simulink model "SGBMDisparity"  (R2021a)
settings: Solver=FixedStepDiscrete  StartTime=0.0  StopTime=simT  FixedStep=1  RelTol=1e-3
PreLoadFcn:
  | DL128 = Simulink.Variant('disparityLevels==128');
  | 
  | DLnot128 = Simulink.Variant('disparityLevels ~= 128');
  | 
  | disparityLevels = 64;
  | 
  | imgRowSize = 480;
  | 
  | imgColSize = 640;
  | 
  | P2 = 200; % Smoothness Penalty Large
  | P1 = 15;  % Smoothness Penalty Small
  | 
  | disparityFactor = 16;
  | 
  | uniquenessRatio = 5;
  | 
  | p = imgColSize - 1;
  | q = imgRowSize * imgColSize -1;
  | r = imgColSize - disparityLevels -1;
  | s = (imgRowSize*(imgColSize-disparityLevels))-1;
  | 
  | simT = 800*525
  | 
  | dtGain = 4;
InitFcn:
  | DL128 = Simulink.Variant('disparityLevels==128');
  | 
  | DLnot128 = Simulink.Variant('disparityLevels ~= 128');
  | 
  | img = imread(get_param('SGBMDisparity/stereoImage','FileName'));
  | 
  | [imgRowSize, imgColSize,chn] = size(img);
  | 
  | P2 = 200; % Smoothness Penalty Large
  | P1 = 15;  % Smoothness Penalty Small
  | 
  | disparityFactor = 16;
  | 
  | uniquenessRatio = str2num(get_param('SGBMDisparity/SGBMHDLAlgorithm/SGBMHDLAlgorithmWorker','UT'));
  | 
  | disparityLevels = str2num(get_param('SGBMDisparity/SGBMHDLAlgorithm/SGBMHDLAlgorithmWorker','DL'));
  | 
  | p = imgColSize - 1;
  | q = imgRowSize * imgColSize -1;
  | r = imgColSize - disparityLevels -1;
  | s = (imgRowSize*(imgColSize-disparityLevels))-1;
  | 
  | if imgRowSize == 720 && imgColSize == 1280
  | simT = 1650*750;
  | elseif imgRowSize == 540 && imgColSize == 960
  | simT = 1050*600;
  | elseif imgRowSize == 480 && imgColSize == 640
  | simT = 800*525;
  | end
  | 
  | %if imgRowSize == 720 && imgColSize == 1280
  | %dtGain = 2;
  | %elseif imgRowSize == 540 && imgColSize == 960
  | %dtGain = 2.6;
  | %elseif imgRowSize == 480 && imgColSize == 640
  | %dtGain = 4;
  | %end
  | 
  | dtGain = 8;
libraries: simulink x331, hdlsllib x113, visionhdlutilities x9, visionhdlio x2, visionsources x1
(part 2 of 6)

== system SGBMDisparity/SGBMHDLAlgorithm/SGBMHDLAlgorithmWorker/DirectionalCost/RightToLeft/InverseRow_ForEach ==
  In : Inport  Partition=on  PartitionDimension=1  PartitionWidth=1  PartitionOffset=0
  busIn : Inport  Port=2
  Bus Selector : BusSelector  OutputSignals=valid,hStart,hEnd,vStart
  Compare To Constant : simulink/Logic and Bit Operations/Compare To Constant  relop===  const=1  OutDataTypeStr=boolean
  Compare To Constant1 : simulink/Logic and Bit Operations/Compare To Constant  relop===  const=1  OutDataTypeStr=boolean
  Compare To Constant3 : simulink/Logic and Bit Operations/Compare To Constant  relop===  const=1  OutDataTypeStr=boolean
  Compare To Constant4 : simulink/Logic and Bit Operations/Compare To Constant  relop===  const=imgColSize-disparityLevels-1  OutDataTypeStr=boolean
  Constant : Constant  Value=0  OutDataTypeStr=boolean  SampleTime=-1
  Constant1 : Constant  Value=0  OutDataTypeStr=boolean  SampleTime=-1
  Delay{1..8} (8 alike) : Delay  DelayLength=1
  For Each : ForEach  DisableCoverage=on
  HDL Counter : hdlsllib/Sources/HDL Counter  CountType=Count limited  CountInit=0  CountStep=1  CountMax=imgColSize-disparityLevels-1  CountFromType=Initial value  CountFrom=0  CountResetPort=on  CountLoadPort=off  CountEnbPort=on  CountDirPort=off  CountHitOutputPort=off  CountDataType=Unsigned  CountWordLen=ceil(log2(imgColSize-disparityLevels-1))  CountFracLen=0  CountSampTime=1
  HDL Counter1 : hdlsllib/Sources/HDL Counter  CountType=Count limited  CountInit=imgColSize-disparityLevels-1  CountStep=1  CountMax=0  CountFromType=Initial value  CountFrom=imgColSize-disparityLevels-1  CountResetPort=on  CountLoadPort=off  CountEnbPort=on  CountDirPort=on  CountHitOutputPort=off  CountDataType=Unsigned  CountWordLen=ceil(log2(imgColSize-disparityLevels-1))  CountFracLen=0  CountSampTime=1
  HDL Counter2 : hdlsllib/Sources/HDL Counter  CountType=Count limited  CountInit=0  CountStep=1  CountMax=1  CountFromType=Initial value  CountFrom=0  CountResetPort=on  CountLoadPort=off  CountEnbPort=on  CountDirPort=off  CountHitOutputPort=off  CountDataType=Unsigned  CountWordLen=1  CountFracLen=0  CountSampTime=1
  HDL Counter3 : hdlsllib/Sources/HDL Counter  CountType=Count limited  CountInit=imgColSize-disparityLevels-1  CountStep=1  CountMax=0  CountFromType=Initial value  CountFrom=imgColSize-disparityLevels-1  CountResetPort=on  CountLoadPort=off  CountEnbPort=on  CountDirPort=on  CountHitOutputPort=off  CountDataType=Unsigned  CountWordLen=ceil(log2(imgColSize-disparityLevels-1))  CountFracLen=0  CountSampTime=1
  HDL Counter4 : hdlsllib/Sources/HDL Counter  CountType=Count limited  CountInit=0  CountStep=1  CountMax=imgColSize-disparityLevels-1  CountFromType=Initial value  CountFrom=0  CountResetPort=on  CountLoadPort=off  CountEnbPort=on  CountDirPort=off  CountHitOutputPort=off  CountDataType=Unsigned  CountWordLen=ceil(log2(imgColSize-disparityLevels-1))  CountFracLen=0  CountSampTime=1
  HDL Counter5 : hdlsllib/Sources/HDL Counter  CountType=Count limited  CountInit=0  CountStep=1  CountMax=1  CountFromType=Initial value  CountFrom=0  CountResetPort=on  CountLoadPort=off  CountEnbPort=on  CountDirPort=off  CountHitOutputPort=off  CountDataType=Unsigned  CountWordLen=1  CountFracLen=0  CountSampTime=1
  HDL Counter6 : hdlsllib/Sources/HDL Counter  CountType=Count limited  CountInit=0  CountStep=1  CountMax=imgColSize-disparityLevels-1  CountFromType=Initial value  CountFrom=0  CountResetPort=on  CountLoadPort=off  CountEnbPort=on  CountDirPort=off  CountHitOutputPort=off  CountDataType=Unsigned  CountWordLen=ceil(log2(imgColSize-disparityLevels-1))  CountFracLen=0  CountSampTime=1
  HDL Counter7 : hdlsllib/Sources/HDL Counter  CountType=Count limited  CountInit=0  CountStep=1  CountMax=1  CountFromType=Initial value  CountFrom=0  CountResetPort=on  CountLoadPort=off  CountEnbPort=on  CountDirPort=off  CountHitOutputPort=off  CountDataType=Unsigned  CountWordLen=2  CountFracLen=0  CountSampTime=1
  Logical Operator : Logic  AllPortsSameDT=off  OutDataTypeStr=boolean
  Logical Operator1 : Logic  Operator=OR  AllPortsSameDT=off  OutDataTypeStr=boolean
  Rd_En : simulink/Logic and Bit Operations/Compare To Constant  relop=<=  const=imgColSize-disparityLevels-1  OutDataTypeStr=boolean
  Simple Dual Port RAM : hdlsllib/HDL RAMs/Simple Dual Port RAM  ram_size=ceil(log2(imgColSize-disparityLevels-1))
      settings: SourceProductBaseCode=SL
  Switch : Switch  Criteria=u2 ~= 0
  Switch1 : Switch  Criteria=u2 ~= 0
  Out : Outport  ConcatenationDimension=1  VectorParamsAs1DForOutWhenUnconnected=off
  valid_Out : Outport  Port=2  ConcatenationDimension=1  VectorParamsAs1DForOutWhenUnconnected=off
  wires:
  Compare To Constant4/1 -> Logical Operator1/2, HDL Counter6/1
  Simple Dual Port RAM/1 -> Out/1
  In/1 -> Delay4/1
  Delay7/1 -> valid_Out/1
  Constant/1 -> HDL Counter1/3
  Logical Operator/1 -> HDL Counter4/2, Delay7/1, HDL Counter3/2
  Compare To Constant/1 -> Switch/2
  Rd_En/1 -> Logical Operator/2
  HDL Counter2/1 -> Compare To Constant/1
  Switch1/1 -> Simple Dual Port RAM/4
  HDL Counter4/1 -> Switch1/3
  Compare To Constant1/1 -> Switch1/2
  HDL Counter/1 -> Switch/1
  Delay3/1 -> HDL Counter7/2, HDL Counter5/2
  HDL Counter7/1 -> Compare To Constant3/1
  Constant1/1 -> HDL Counter3/3
  Delay1/1 -> Simple Dual Port RAM/3, HDL Counter1/2, HDL Counter/2
  HDL Counter6/1 -> Rd_En/1, Compare To Constant4/1
  Compare To Constant3/1 -> Logical Operator/1, HDL Counter6/2
  HDL Counter3/1 -> Switch1/1
  Switch/1 -> Simple Dual Port RAM/2
  HDL Counter5/1 -> Compare To Constant1/1
  HDL Counter1/1 -> Switch/3
  Delay2/1 -> Simple Dual Port RAM/1
  Bus Selector/1 -> Delay5/1  "<valid>"
  busIn/1 -> Bus Selector/1
  Bus Selector/2 -> Delay6/1  "<hStart>"
  Bus Selector/3 -> Delay8/1  "<hEnd>"
  Logical Operator1/1 -> HDL Counter7/1
  Bus Selector/4 -> Logical Operator1/1, HDL Counter5/1, HDL Counter2/1, HDL Counter4/1, HDL Counter3/1, HDL Counter/1, HDL Counter1/1  "<vStart>"
  Delay4/1 -> Delay2/1
  Delay5/1 -> Delay1/1
  Delay6/1 -> HDL Counter2/2
  Delay8/1 -> Delay3/1

== system SGBMDisparity/SGBMHDLAlgorithm/SGBMHDLAlgorithmWorker/DirectionalCost/RightToLeft/pixelBusGenerator ==
  validIn : Inport
  Horizontal : hdlsllib/Sources/HDL Counter  CountType=Count limited  CountInit=0  CountStep=1  CountMax=hEnd  CountFromType=Initial value  CountFrom=0  CountResetPort=off  CountLoadPort=off  CountEnbPort=on  CountDirPort=off  CountHitOutputPort=off  CountDataType=Unsigned  CountWordLen=ceil(log2(hEnd))  CountFracLen=0  CountSampTime=1
  Logical Operator{3..6} (4 alike) : Logic  AllPortsSameDT=off  OutDataTypeStr=boolean
  Pixel Control Bus Creator : visionhdlutilities/Pixel Control Bus Creator
      settings: SourceProductBaseCode=VT
  Vertical : hdlsllib/Sources/HDL Counter  CountType=Count limited  CountInit=0  CountStep=1  CountMax=vEnd  CountFromType=Initial value  CountFrom=0  CountResetPort=off  CountLoadPort=off  CountEnbPort=on  CountDirPort=off  CountHitOutputPort=off  CountDataType=Unsigned  CountWordLen=ceil(log2(vEnd))  CountFracLen=0  CountSampTime=1
  hEnd : simulink/Logic and Bit Operations/Compare To Constant  relop===  const=hEnd  OutDataTypeStr=boolean
  hStart : simulink/Logic and Bit Operations/Compare To Constant  relop===  const=0  OutDataTypeStr=boolean
  vEnd : simulink/Logic and Bit Operations/Compare To Constant  relop===  const=vEnd  OutDataTypeStr=boolean
  vStart : simulink/Logic and Bit Operations/Compare To Constant  relop===  const=0  OutDataTypeStr=boolean
  busOut : Outport  VectorParamsAs1DForOutWhenUnconnected=off
  wires:
  validIn/1 -> Pixel Control Bus Creator/5, Vertical/1, Logical Operator4/1, Logical Operator5/1, Logical Operator6/1, Logical Operator3/1, Horizontal/1
  Horizontal/1 -> hEnd/1, hStart/1
  hEnd/1 -> Logical Operator4/2
  Vertical/1 -> vStart/1, vEnd/1
  vStart/1 -> Logical Operator5/2
  vEnd/1 -> Logical Operator6/2
  Logical Operator5/1 -> Pixel Control Bus Creator/3
  Logical Operator3/1 -> Pixel Control Bus Creator/1
  Logical Operator4/1 -> Pixel Control Bus Creator/2
  hStart/1 -> Logical Operator3/2
  Logical Operator6/1 -> Pixel Control Bus Creator/4
  Pixel Control Bus Creator/1 -> busOut/1

== system SGBMDisparity/SGBMHDLAlgorithm/SGBMHDLAlgorithmWorker/DirectionalCost/RightToLeft/rlSubsystem ==
  enable : Inport
  matchCostIn : Inport  Port=2
  Enable : EnablePort
  Delay : Delay  DelayLength=1
  For Each Subsystem : Subsystem  TreatAsAtomicUnit=on
  MinMax1 : MinMax  ZeroCross=off
  Signal Specification : SignalSpecification  Dimensions=disparityLevels
  Switch32 : Switch  Criteria=u2 ~= 0
  d+1 : Subsystem
  d-1 : Subsystem
  minCostPath : Subsystem  TreatAsAtomicUnit=on
  Out1 : Outport  InitialOutput=0  VectorParamsAs1DForOutWhenUnconnected=off
  wires:
  matchCostIn/1 -> minCostPath/1(Matching_Cost)
  Delay/1 -> minCostPath/2(prev_cost_d), d+1/1(prev_cost_d), d-1/1(prev_cost_d), MinMax1/1
  For Each Subsystem/1(Out1) -> Switch32/3
  MinMax1/1 -> minCostPath/5(min_prev_cost)
  Signal Specification/1 -> For Each Subsystem/1(In1)
  d+1/1(prev_cost_d+1) -> minCostPath/4(prev_cost_d+1)
  d-1/1(prev_cost_d-1) -> minCostPath/3(prev_cost_d-1)
  Switch32/1 -> Delay/1
  minCostPath/1(curr_cost) -> Out1/1, Switch32/1, Signal Specification/1
  enable/1 -> Switch32/2

== system SGBMDisparity/SGBMHDLAlgorithm/SGBMHDLAlgorithmWorker/DirectionalCost/TopLeftToBottomRight/tlbrSubsystem ==
  enable : Inport
  matchCostIn : Inport  Port=2
  Enable : EnablePort
  Delay1 : Delay  DelayLength=1
  Delay2 : Delay  DelayLength=imgColSize-disparityLevels
  Delay4 : Delay  DelayLength=1
  For Each Subsystem : Subsystem  TreatAsAtomicUnit=on
  Min : MinMax
  Signal Specification : SignalSpecification  Dimensions=disparityLevels
  Switch1 : Switch  Criteria=u2 ~= 0
  d+2 : Subsystem
  d-2 : Subsystem
  minCostPath : Subsystem  TreatAsAtomicUnit=on
  tlbrCost : Outport  InitialOutput=0  VectorParamsAs1DForOutWhenUnconnected=off
  wires:
  d+2/1(prev_cost_d+1) -> minCostPath/4(prev_cost_d+1)
  Delay2/1 -> Min/1, Delay4/1
  Min/1 -> Delay1/1
  For Each Subsystem/1(Out1) -> Switch1/3
  Switch1/1 -> Delay2/1
  Signal Specification/1 -> For Each Subsystem/1(In1)
  Delay1/1 -> minCostPath/5(min_prev_cost)
  d-2/1(prev_cost_d-1) -> minCostPath/3(prev_cost_d-1)
  enable/1 -> Switch1/2
  Delay4/1 -> d+2/1(prev_cost_d), d-2/1(prev_cost_d), minCostPath/2(prev_cost_d)
  minCostPath/1(curr_cost) -> tlbrCost/1, Switch1/1, Signal Specification/1
  matchCostIn/1 -> minCostPath/1(Matching_Cost)

== system SGBMDisparity/SGBMHDLAlgorithm/SGBMHDLAlgorithmWorker/DirectionalCost/TopRightToBottomLeft/trblSubsystem ==
  enable : Inport
  matchCostIn : Inport  Port=2
  Enable : EnablePort
  Delay1 : Delay  DelayLength=1
  Delay20 : Delay  DelayLength=imgColSize-disparityLevels-2
  Delay4 : Delay  DelayLength=1
  For Each Subsystem : Subsystem  TreatAsAtomicUnit=on
  Min : MinMax
  Signal Specification : SignalSpecification  Dimensions=disparityLevels
  Switch1 : Switch  Criteria=u2 ~= 0
  d+2 : Subsystem
  d-2 : Subsystem
  minCostPath : Subsystem  TreatAsAtomicUnit=on
  trblCost : Outport  InitialOutput=0  VectorParamsAs1DForOutWhenUnconnected=off
  wires:
  Delay1/1 -> minCostPath/5(min_prev_cost)
  Min/1 -> Delay1/1
  Delay20/1 -> Min/1, Delay4/1
  d+2/1(prev_cost_d+1) -> minCostPath/4(prev_cost_d+1)
  minCostPath/1(curr_cost) -> trblCost/1, Switch1/1, Signal Specification/1
  For Each Subsystem/1(Out1) -> Switch1/3
  d-2/1(prev_cost_d-1) -> minCostPath/3(prev_cost_d-1)
  Switch1/1 -> Delay20/1
  Delay4/1 -> d+2/1(prev_cost_d), d-2/1(prev_cost_d), minCostPath/2(prev_cost_d)
  matchCostIn/1 -> minCostPath/1(Matching_Cost)
  Signal Specification/1 -> For Each Subsystem/1(In1)
  enable/1 -> Switch1/2

== system SGBMDisparity/SGBMHDLAlgorithm/SGBMHDLAlgorithmWorker/DirectionalCost/TopToBottom/tbSubsystem ==
  enable : Inport
  matchCostIn : Inport  Port=2
  Enable : EnablePort
  Delay1 : Delay  DelayLength=1
  Delay2 : Delay  DelayLength=imgColSize-disparityLevels-1
  Delay4 : Delay  DelayLength=1
  For Each Subsystem : Subsystem  TreatAsAtomicUnit=on
  Min : MinMax
  Signal Specification : SignalSpecification  Dimensions=disparityLevels
  Switch1 : Switch  Criteria=u2 ~= 0
  d+1 : Subsystem
  d-1 : Subsystem
  minCostPath : Subsystem  TreatAsAtomicUnit=on
  tbCost : Outport  InitialOutput=0  VectorParamsAs1DForOutWhenUnconnected=off
  wires:
  d+1/1(prev_cost_d+1) -> minCostPath/4(prev_cost_d+1)
  d-1/1(prev_cost_d-1) -> minCostPath/3(prev_cost_d-1)
  minCostPath/1(curr_cost) -> Switch1/1, Signal Specification/1, tbCost/1
  Delay4/1 -> d+1/1(prev_cost_d), d-1/1(prev_cost_d), minCostPath/2(prev_cost_d)
  For Each Subsystem/1(Out1) -> Switch1/3
  Delay2/1 -> Min/1, Delay4/1
  Min/1 -> Delay1/1
  enable/1 -> Switch1/2
  Switch1/1 -> Delay2/1
  Signal Specification/1 -> For Each Subsystem/1(In1)
  Delay1/1 -> minCostPath/5(min_prev_cost)
  matchCostIn/1 -> minCostPath/1(Matching_Cost)

== system SGBMDisparity/SGBMHDLAlgorithm/SGBMHDLAlgorithmWorker/MatchingCost/CensusTransform/ctLogic ==
  pixelIn : Inport
  Enable : EnablePort
  Bit Concat : hdlsllib/Logic and Bit Operations/Bit Concat  numInputs=31
  Delay{1,3..4,6,12} (5 alike) : Delay  DelayLength=9
  Delay{2,9..11,13..14} (6 alike) : Delay  DelayLength=imgColSize-1
  Delay5 : Delay  DelayLength=1
  Delay7 : Delay  DelayLength=4
  Delay8 : Delay  DelayLength=4
  Demux : Demux  Outputs=9
  Demux1 : Demux  Outputs=9
  Demux2 : Demux  Outputs=9
  Demux3 : Demux
  For Each Subsystem : Subsystem  TreatAsAtomicUnit=on
  For Each Subsystem1 : Subsystem  TreatAsAtomicUnit=on
  For Each Subsystem2 : Subsystem  TreatAsAtomicUnit=on
  For Each Subsystem3 : Subsystem  TreatAsAtomicUnit=on
  Tapped Delay : simulink/Discrete/Tapped Delay  vinit=0.0  samptime=-1  NumDelays=8  DelayOrder=Newest  includeCurrent=on
  Tapped Delay1 : simulink/Discrete/Tapped Delay  vinit=0.0  samptime=-1  NumDelays=8  DelayOrder=Newest  includeCurrent=on
  Tapped Delay2 : simulink/Discrete/Tapped Delay  vinit=0.0  samptime=-1  NumDelays=8  DelayOrder=Newest  includeCurrent=on
  Tapped Delay3 : simulink/Discrete/Tapped Delay  vinit=0.0  samptime=-1  NumDelays=3  DelayOrder=Newest  includeCurrent=on
  Tapped Delay4 : simulink/Discrete/Tapped Delay  vinit=0.0  samptime=-1  NumDelays=3  DelayOrder=Oldest  includeCurrent=on
  Tapped Delay5 : simulink/Discrete/Tapped Delay  vinit=0.0  samptime=-1  NumDelays=8  DelayOrder=Oldest  includeCurrent=on
  Tapped Delay6 : simulink/Discrete/Tapped Delay  vinit=0.0  samptime=-1  NumDelays=8  DelayOrder=Oldest  includeCurrent=on
  Tapped Delay7 : simulink/Discrete/Tapped Delay  vinit=0.0  samptime=-1  NumDelays=8  DelayOrder=Oldest  includeCurrent=on
  resultOut : Outport  InitialOutput=0  VectorParamsAs1DForOutWhenUnconnected=off
  wires:
  Demux/2 -> Bit Concat/2
  Demux/7 -> Bit Concat/7
  Demux2/3 -> Bit Concat/21
  Demux1/1 -> Bit Concat/10
  Delay5/1 -> Delay7/1, Tapped Delay4/1
  For Each Subsystem/1(Out1) -> Demux/1
  Delay13/1 -> Delay8/1, Tapped Delay3/1
  Delay7/1 -> Delay10/1
  For Each Subsystem2/1(Out1) -> Demux3/1
  Tapped Delay5/1 -> For Each Subsystem1/1(In1)
  Demux3/2 -> Bit Concat/29
  Tapped Delay6/1 -> For Each Subsystem3/1(In1)
  Delay1/1 -> Delay2/1
  Demux2/8 -> Bit Concat/26
  Delay3/1 -> Delay11/1
  pixelIn/1 -> Tapped Delay/1, Delay1/1
  Demux1/4 -> Bit Concat/13
  Demux1/6 -> Bit Concat/15
  Demux1/3 -> Bit Concat/12
  Demux2/5 -> Bit Concat/23
  Delay6/1 -> Delay13/1
  Tapped Delay3/1 -> For Each Subsystem2/2(In2)
  Demux/4 -> Bit Concat/4
  Tapped Delay4/1 -> For Each Subsystem2/1(In1)
  Delay2/1 -> Delay3/1, Tapped Delay1/1
  Delay9/1 -> Delay12/1, Tapped Delay6/1
  Demux3/1 -> Bit Concat/28
  Demux2/2 -> Bit Concat/20
  Demux/6 -> Bit Concat/6
  For Each Subsystem3/1(Out1) -> Demux1/1
  Tapped Delay1/1 -> For Each Subsystem3/2(In2)
  Tapped Delay7/1 -> For Each Subsystem/1(In1)
  Demux1/2 -> Bit Concat/11
  Demux2/4 -> Bit Concat/22
  Demux3/4 -> Bit Concat/31
  For Each Subsystem1/1(Out1) -> Demux2/1
  Demux/8 -> Bit Concat/8
  Demux/9 -> Bit Concat/9
  Demux/5 -> Bit Concat/5
  Demux3/3 -> Bit Concat/30
  Demux1/5 -> Bit Concat/14
  Demux2/9 -> Bit Concat/27
  Tapped Delay/1 -> For Each Subsystem/2(In2)
  Delay11/1 -> Delay6/1, Tapped Delay2/1
  Delay10/1 -> Delay4/1, Tapped Delay5/1
  Demux2/7 -> Bit Concat/25
  Demux/3 -> Bit Concat/3
  Tapped Delay2/1 -> For Each Subsystem1/2(In2)
  Demux1/7 -> Bit Concat/16
  Demux1/8 -> Bit Concat/17
  Demux2/6 -> Bit Concat/24
  Delay8/1 -> Delay5/1
  Bit Concat/1 -> resultOut/1
  Demux/1 -> Bit Concat/1
  Delay14/1 -> Tapped Delay7/1
  Delay12/1 -> Delay14/1
  Demux1/9 -> Bit Concat/18
  Delay4/1 -> Delay9/1
  Demux2/1 -> Bit Concat/19

== system SGBMDisparity/SGBMHDLAlgorithm/SGBMHDLAlgorithmWorker/MatchingCost/CensusTransform/dataAligner ==
  dataIn : Inport
  busIn : Inport  Port=2
  Bus Selector : BusSelector  OutputSignals=vStart,valid,hEnd
  CC1 : simulink/Logic and Bit Operations/Compare To Constant  relop===  const=imgColSize-1  OutDataTypeStr=boolean
  CC5 : simulink/Logic and Bit Operations/Compare To Constant  relop===  const=1  OutDataTypeStr=boolean
  Delay{,1..3} (4 alike) : Delay  DelayLength=1
  HDL Counter : hdlsllib/Sources/HDL Counter  CountType=Count limited  CountInit=0  CountStep=1  CountMax=imgColSize-1  CountFromType=Initial value  CountFrom=0  CountResetPort=on  CountLoadPort=off  CountEnbPort=on  CountDirPort=off  CountHitOutputPort=off  CountDataType=Unsigned  CountWordLen=ceil(log2(imgColSize))  CountFracLen=0  CountSampTime=1
  HDL Counter1 : hdlsllib/Sources/HDL Counter  CountType=Count limited  CountInit=0  CountStep=1  CountMax=imgColSize-1  CountFromType=Initial value  CountFrom=0  CountResetPort=on  CountLoadPort=off  CountEnbPort=on  CountDirPort=off  CountHitOutputPort=off  CountDataType=Unsigned  CountWordLen=ceil(log2(imgColSize))  CountFracLen=0  CountSampTime=1
  HDLC3 : hdlsllib/Sources/HDL Counter  CountType=Count limited  CountInit=0  CountStep=1  CountMax=3  CountFromType=Initial value  CountFrom=0  CountResetPort=on  CountLoadPort=off  CountEnbPort=on  CountDirPort=off  CountHitOutputPort=off  CountDataType=Unsigned  CountWordLen=2  CountFracLen=0  CountSampTime=1
  Simple Dual Port RAM : hdlsllib/HDL RAMs/Simple Dual Port RAM  ram_size=ceil(log2(imgColSize))
      settings: SourceProductBaseCode=SL
  pixelBusGenerator : Subsystem  mask{hEnd=p, vEnd=q}
      mask prompts: hEnd "hEnd Count"; vEnd "vEnd Count"
      mask DialogControl DescGroupVar Prompt: Counter Values
  dataOut : Outport  VectorParamsAs1DForOutWhenUnconnected=off
  busOut : Outport  Port=2  VectorParamsAs1DForOutWhenUnconnected=off
  wires:
  HDL Counter1/1 -> CC1/1, Simple Dual Port RAM/4
  CC5/1 -> Delay/1, HDL Counter1/2
  HDL Counter/1 -> Simple Dual Port RAM/2
  dataIn/1 -> Delay1/1
  Simple Dual Port RAM/1 -> dataOut/1
  busIn/1 -> Bus Selector/1
  Bus Selector/1 -> HDL Counter1/1, HDL Counter/1  "<vStart>"
  Bus Selector/2 -> Delay2/1  "<valid>"
  HDLC3/1 -> CC5/1
  Bus Selector/3 -> Delay3/1  "<hEnd>"
  CC1/1 -> HDLC3/1
  Delay/1 -> pixelBusGenerator/1(validIn)
  pixelBusGenerator/1(busOut) -> busOut/1
  Delay1/1 -> Simple Dual Port RAM/1
  Delay2/1 -> Simple Dual Port RAM/3, HDL Counter/2
  Delay3/1 -> HDLC3/2

== system SGBMDisparity/SGBMHDLAlgorithm/SGBMHDLAlgorithmWorker/MatchingCost/CensusTransform/validLogic ==
  validIn : Inport
  reset : Inport  Port=2
  CC : simulink/Logic and Bit Operations/Compare To Constant  relop===  const=imgColSize+7  OutDataTypeStr=boolean
  CC1 : simulink/Logic and Bit Operations/Compare To Constant  relop=>  const=7  OutDataTypeStr=boolean
  CC2 : simulink/Logic and Bit Operations/Compare To Constant  relop=<=  const=imgColSize+7  OutDataTypeStr=boolean
  CC3 : simulink/Logic and Bit Operations/Compare To Constant  relop=>  const=5  OutDataTypeStr=boolean
  CC4 : simulink/Logic and Bit Operations/Compare To Constant  relop=<=  const=imgRowSize+5  OutDataTypeStr=boolean
  HDL Counter : hdlsllib/Sources/HDL Counter  CountType=Count limited  CountInit=0  CountStep=1  CountMax=imgColSize+7  CountFromType=Initial value  CountFrom=0  CountResetPort=on  CountLoadPort=off  CountEnbPort=on  CountDirPort=off  CountHitOutputPort=off  CountDataType=Unsigned  CountWordLen=ceil(log2(imgColSize+7))  CountFracLen=0  CountSampTime=1
  HDL Counter1 : hdlsllib/Sources/HDL Counter  CountType=Count limited  CountInit=0  CountStep=1  CountMax=imgRowSize+5  CountFromType=Initial value  CountFrom=0  CountResetPort=on  CountLoadPort=off  CountEnbPort=on  CountDirPort=off  CountHitOutputPort=off  CountDataType=Unsigned  CountWordLen=ceil(log2(imgRowSize+5))  CountFracLen=0  CountSampTime=1
  LO : Logic  AllPortsSameDT=off  OutDataTypeStr=boolean
  LO1 : Logic  Inputs=5  AllPortsSameDT=off  OutDataTypeStr=boolean
  pixelBusGenerator : Subsystem  mask{hEnd=p, vEnd=q}
      mask prompts: hEnd "hEnd Count"; vEnd "vEnd Count"
      mask DialogControl DescGroupVar Prompt: Counter Values
  busOut : Outport  VectorParamsAs1DForOutWhenUnconnected=off
  wires:
  HDL Counter/1 -> CC2/1, CC1/1, CC/1
  CC/1 -> LO/1
  LO/1 -> HDL Counter1/2
  validIn/1 -> LO1/5, LO/2, HDL Counter/2
  HDL Counter1/1 -> CC4/1, CC3/1
  CC1/1 -> LO1/3
  CC2/1 -> LO1/4
  CC3/1 -> LO1/1
  CC4/1 -> LO1/2
  reset/1 -> HDL Counter1/1, HDL Counter/1
  LO1/1 -> pixelBusGenerator/1(validIn)
  pixelBusGenerator/1(busOut) -> busOut/1

== system SGBMDisparity/SGBMHDLAlgorithm/SGBMHDLAlgorithmWorker/MatchingCost/CensusTransform/zeroPadding ==
  pixelIn : Inport
  ctrlIn : Inport  Port=2
  Bus Selector : BusSelector  OutputSignals=valid,hStart,vStart
  CC5 : simulink/Logic and Bit Operations/Compare To Constant  relop===  const=1  OutDataTypeStr=boolean
  Constant : Constant  Value=0  VectorParams1D=off  OutDataTypeStr=uint8  SampleTime=-1
  Delay{,1..6,14} (8 alike) : Delay  DelayLength=1
  FIFO : Subsystem
  HDLC3 : hdlsllib/Sources/HDL Counter  CountType=Count limited  CountInit=0  CountStep=1  CountMax=3  CountFromType=Initial value  CountFrom=0  CountResetPort=on  CountLoadPort=off  CountEnbPort=on  CountDirPort=off  CountHitOutputPort=off  CountDataType=Unsigned  CountWordLen=2  CountFracLen=0  CountSampTime=1
  Logical Operator : Logic  Operator=OR  AllPortsSameDT=off  OutDataTypeStr=boolean
  Logical Operator1 : Logic  AllPortsSameDT=off  OutDataTypeStr=boolean
  Logical Operator2 : Logic  AllPortsSameDT=off  OutDataTypeStr=boolean
  Logical Operator3 : Logic  Operator=NOT  AllPortsSameDT=off  OutDataTypeStr=boolean
  Logical Operator4 : Logic  Operator=OR  Inputs=3  AllPortsSameDT=off  OutDataTypeStr=boolean
  Logical Operator5 : Logic  AllPortsSameDT=off  OutDataTypeStr=boolean
  Switch : Switch  Criteria=u2 ~= 0  ZeroCross=off
  popSubsystem : Subsystem
  pixelOut : Outport  VectorParamsAs1DForOutWhenUnconnected=off
  validOut : Outport  Port=2  VectorParamsAs1DForOutWhenUnconnected=off
  resetOut : Outport  Port=3  VectorParamsAs1DForOutWhenUnconnected=off
  wires:
  FIFO/1(dataOut) -> Switch/1
  Bus Selector/2 -> Delay4/1  "<hStart>"
  Bus Selector/3 -> resetOut/1, Logical Operator4/1, FIFO/4(Reset), Logical Operator/2, Delay5/1  "<vStart>"
  Switch/1 -> pixelOut/1
  FIFO/2(empty) -> Logical Operator3/1
  Bus Selector/1 -> Delay/1  "<valid>"
  Delay1/1 -> validOut/1
  Delay14/1 -> Switch/2
  Constant/1 -> Switch/3
  ctrlIn/1 -> Bus Selector/1
  pixelIn/1 -> Delay3/1
  Logical Operator2/1 -> FIFO/3(Pop), Delay14/1
  popSubsystem/2(pop) -> Logical Operator2/1
  Logical Operator4/1 -> Logical Operator5/1, popSubsystem/Enable
  Logical Operator3/1 -> Logical Operator4/2, Logical Operator2/2
  popSubsystem/3(lastRowOut) -> Delay2/1
  Logical Operator5/1 -> Delay1/1
  HDLC3/1 -> CC5/1
  Logical Operator1/1 -> HDLC3/2
  CC5/1 -> Logical Operator5/2, popSubsystem/1(enable)
  Delay2/1 -> Logical Operator4/3
  Delay/1 -> FIFO/2(Push)
  Delay3/1 -> FIFO/1(dataIn)
  Delay4/1 -> Logical Operator1/1
  Logical Operator/1 -> popSubsystem/2(reset), HDLC3/1
  popSubsystem/1(done) -> Delay6/1
  Delay5/1 -> Logical Operator1/2
  Delay6/1 -> Logical Operator/1

== system SGBMDisparity/SGBMHDLAlgorithm/SGBMHDLAlgorithmWorker/MatchingCost/CensusTransform1/ctLogic ==
  pixelIn : Inport
  Enable : EnablePort
  Bit Concat : hdlsllib/Logic and Bit Operations/Bit Concat  numInputs=31
  Delay{1,3..4,6,12} (5 alike) : Delay  DelayLength=9
  Delay{2,9..11,13..14} (6 alike) : Delay  DelayLength=imgColSize-1
  Delay5 : Delay  DelayLength=1
  Delay7 : Delay  DelayLength=4
  Delay8 : Delay  DelayLength=4
  Demux : Demux  Outputs=9
  Demux1 : Demux  Outputs=9
  Demux2 : Demux  Outputs=9
  Demux3 : Demux
  For Each Subsystem : Subsystem  TreatAsAtomicUnit=on
  For Each Subsystem1 : Subsystem  TreatAsAtomicUnit=on
  For Each Subsystem2 : Subsystem  TreatAsAtomicUnit=on
  For Each Subsystem3 : Subsystem  TreatAsAtomicUnit=on
  Tapped Delay : simulink/Discrete/Tapped Delay  vinit=0.0  samptime=-1  NumDelays=8  DelayOrder=Newest  includeCurrent=on
  Tapped Delay1 : simulink/Discrete/Tapped Delay  vinit=0.0  samptime=-1  NumDelays=8  DelayOrder=Newest  includeCurrent=on
  Tapped Delay2 : simulink/Discrete/Tapped Delay  vinit=0.0  samptime=-1  NumDelays=8  DelayOrder=Newest  includeCurrent=on
  Tapped Delay3 : simulink/Discrete/Tapped Delay  vinit=0.0  samptime=-1  NumDelays=3  DelayOrder=Newest  includeCurrent=on
  Tapped Delay4 : simulink/Discrete/Tapped Delay  vinit=0.0  samptime=-1  NumDelays=3  DelayOrder=Oldest  includeCurrent=on
  Tapped Delay5 : simulink/Discrete/Tapped Delay  vinit=0.0  samptime=-1  NumDelays=8  DelayOrder=Oldest  includeCurrent=on
  Tapped Delay6 : simulink/Discrete/Tapped Delay  vinit=0.0  samptime=-1  NumDelays=8  DelayOrder=Oldest  includeCurrent=on
  Tapped Delay7 : simulink/Discrete/Tapped Delay  vinit=0.0  samptime=-1  NumDelays=8  DelayOrder=Oldest  includeCurrent=on
  resultOut : Outport  InitialOutput=0  VectorParamsAs1DForOutWhenUnconnected=off
  wires:
  Demux/2 -> Bit Concat/2
  Demux/7 -> Bit Concat/7
  Demux2/3 -> Bit Concat/21
  Demux1/1 -> Bit Concat/10
  Delay5/1 -> Delay7/1, Tapped Delay4/1
  For Each Subsystem/1(Out1) -> Demux/1
  Delay13/1 -> Delay8/1, Tapped Delay3/1
  Delay7/1 -> Delay10/1
  For Each Subsystem2/1(Out1) -> Demux3/1
  Tapped Delay5/1 -> For Each Subsystem1/1(In1)
  Demux3/2 -> Bit Concat/29
  Tapped Delay6/1 -> For Each Subsystem3/1(In1)
  Delay1/1 -> Delay2/1
  Demux2/8 -> Bit Concat/26
  Delay3/1 -> Delay11/1
  pixelIn/1 -> Tapped Delay/1, Delay1/1
  Demux1/4 -> Bit Concat/13
  Demux1/6 -> Bit Concat/15
  Demux1/3 -> Bit Concat/12
  Demux2/5 -> Bit Concat/23
  Delay6/1 -> Delay13/1
  Tapped Delay3/1 -> For Each Subsystem2/2(In2)
  Demux/4 -> Bit Concat/4
  Tapped Delay4/1 -> For Each Subsystem2/1(In1)
  Delay2/1 -> Delay3/1, Tapped Delay1/1
  Delay9/1 -> Delay12/1, Tapped Delay6/1
  Demux3/1 -> Bit Concat/28
  Demux2/2 -> Bit Concat/20
  Demux/6 -> Bit Concat/6
  For Each Subsystem3/1(Out1) -> Demux1/1
  Tapped Delay1/1 -> For Each Subsystem3/2(In2)
  Tapped Delay7/1 -> For Each Subsystem/1(In1)
  Demux1/2 -> Bit Concat/11
  Demux2/4 -> Bit Concat/22
  Demux3/4 -> Bit Concat/31
  For Each Subsystem1/1(Out1) -> Demux2/1
  Demux/8 -> Bit Concat/8
  Demux/9 -> Bit Concat/9
  Demux/5 -> Bit Concat/5
  Demux3/3 -> Bit Concat/30
  Demux1/5 -> Bit Concat/14
  Demux2/9 -> Bit Concat/27
  Tapped Delay/1 -> For Each Subsystem/2(In2)
  Delay11/1 -> Delay6/1, Tapped Delay2/1
  Delay10/1 -> Delay4/1, Tapped Delay5/1
  Demux2/7 -> Bit Concat/25
  Demux/3 -> Bit Concat/3
  Tapped Delay2/1 -> For Each Subsystem1/2(In2)
  Demux1/7 -> Bit Concat/16
  Demux1/8 -> Bit Concat/17
  Demux2/6 -> Bit Concat/24
  Delay8/1 -> Delay5/1
  Bit Concat/1 -> resultOut/1
  Demux/1 -> Bit Concat/1
  Delay14/1 -> Tapped Delay7/1
  Delay12/1 -> Delay14/1
  Demux1/9 -> Bit Concat/18
  Delay4/1 -> Delay9/1
  Demux2/1 -> Bit Concat/19

== system SGBMDisparity/SGBMHDLAlgorithm/SGBMHDLAlgorithmWorker/MatchingCost/CensusTransform1/dataAligner ==
  dataIn : Inport
  busIn : Inport  Port=2
  Bus Selector : BusSelector  OutputSignals=vStart,valid,hEnd
  CC1 : simulink/Logic and Bit Operations/Compare To Constant  relop===  const=imgColSize-1  OutDataTypeStr=boolean
  CC5 : simulink/Logic and Bit Operations/Compare To Constant  relop===  const=1  OutDataTypeStr=boolean
  Delay{,1..3} (4 alike) : Delay  DelayLength=1
  HDL Counter : hdlsllib/Sources/HDL Counter  CountType=Count limited  CountInit=0  CountStep=1  CountMax=imgColSize-1  CountFromType=Initial value  CountFrom=0  CountResetPort=on  CountLoadPort=off  CountEnbPort=on  CountDirPort=off  CountHitOutputPort=off  CountDataType=Unsigned  CountWordLen=ceil(log2(imgColSize))  CountFracLen=0  CountSampTime=1
  HDL Counter1 : hdlsllib/Sources/HDL Counter  CountType=Count limited  CountInit=0  CountStep=1  CountMax=imgColSize-1  CountFromType=Initial value  CountFrom=0  CountResetPort=on  CountLoadPort=off  CountEnbPort=on  CountDirPort=off  CountHitOutputPort=off  CountDataType=Unsigned  CountWordLen=ceil(log2(imgColSize))  CountFracLen=0  CountSampTime=1
  HDLC3 : hdlsllib/Sources/HDL Counter  CountType=Count limited  CountInit=0  CountStep=1  CountMax=3  CountFromType=Initial value  CountFrom=0  CountResetPort=on  CountLoadPort=off  CountEnbPort=on  CountDirPort=off  CountHitOutputPort=off  CountDataType=Unsigned  CountWordLen=2  CountFracLen=0  CountSampTime=1
  Simple Dual Port RAM : hdlsllib/HDL RAMs/Simple Dual Port RAM  ram_size=ceil(log2(imgColSize))
      settings: SourceProductBaseCode=SL
  pixelBusGenerator : Subsystem  mask{hEnd=p, vEnd=q}
      mask prompts: hEnd "hEnd Count"; vEnd "vEnd Count"
      mask DialogControl DescGroupVar Prompt: Counter Values
  dataOut : Outport  VectorParamsAs1DForOutWhenUnconnected=off
  busOut : Outport  Port=2  VectorParamsAs1DForOutWhenUnconnected=off
  wires:
  HDL Counter1/1 -> CC1/1, Simple Dual Port RAM/4
  CC5/1 -> Delay/1, HDL Counter1/2
  HDL Counter/1 -> Simple Dual Port RAM/2
  dataIn/1 -> Delay1/1
  Simple Dual Port RAM/1 -> dataOut/1
  busIn/1 -> Bus Selector/1
  Bus Selector/1 -> HDL Counter1/1, HDL Counter/1  "<vStart>"
  Bus Selector/2 -> Delay2/1  "<valid>"
  HDLC3/1 -> CC5/1
  Bus Selector/3 -> Delay3/1  "<hEnd>"
  CC1/1 -> HDLC3/1
  Delay/1 -> pixelBusGenerator/1(validIn)
  pixelBusGenerator/1(busOut) -> busOut/1
  Delay1/1 -> Simple Dual Port RAM/1
  Delay2/1 -> Simple Dual Port RAM/3, HDL Counter/2
  Delay3/1 -> HDLC3/2

== system SGBMDisparity/SGBMHDLAlgorithm/SGBMHDLAlgorithmWorker/MatchingCost/CensusTransform1/validLogic ==
  validIn : Inport
  reset : Inport  Port=2
  CC : simulink/Logic and Bit Operations/Compare To Constant  relop===  const=imgColSize+7  OutDataTypeStr=boolean
  CC1 : simulink/Logic and Bit Operations/Compare To Constant  relop=>  const=7  OutDataTypeStr=boolean
  CC2 : simulink/Logic and Bit Operations/Compare To Constant  relop=<=  const=imgColSize+7  OutDataTypeStr=boolean
  CC3 : simulink/Logic and Bit Operations/Compare To Constant  relop=>  const=5  OutDataTypeStr=boolean
  CC4 : simulink/Logic and Bit Operations/Compare To Constant  relop=<=  const=imgRowSize+5  OutDataTypeStr=boolean
  HDL Counter : hdlsllib/Sources/HDL Counter  CountType=Count limited  CountInit=0  CountStep=1  CountMax=imgColSize+7  CountFromType=Initial value  CountFrom=0  CountResetPort=on  CountLoadPort=off  CountEnbPort=on  CountDirPort=off  CountHitOutputPort=off  CountDataType=Unsigned  CountWordLen=ceil(log2(imgColSize+7))  CountFracLen=0  CountSampTime=1
  HDL Counter1 : hdlsllib/Sources/HDL Counter  CountType=Count limited  CountInit=0  CountStep=1  CountMax=imgRowSize+5  CountFromType=Initial value  CountFrom=0  CountResetPort=on  CountLoadPort=off  CountEnbPort=on  CountDirPort=off  CountHitOutputPort=off  CountDataType=Unsigned  CountWordLen=ceil(log2(imgRowSize+5))  CountFracLen=0  CountSampTime=1
  LO : Logic  AllPortsSameDT=off  OutDataTypeStr=boolean
  LO1 : Logic  Inputs=5  AllPortsSameDT=off  OutDataTypeStr=boolean
  pixelBusGenerator : Subsystem  mask{hEnd=p, vEnd=q}
      mask prompts: hEnd "hEnd Count"; vEnd "vEnd Count"
      mask DialogControl DescGroupVar Prompt: Counter Values
  busOut : Outport  VectorParamsAs1DForOutWhenUnconnected=off
  wires:
  HDL Counter/1 -> CC2/1, CC1/1, CC/1
  CC/1 -> LO/1
  LO/1 -> HDL Counter1/2
  validIn/1 -> LO1/5, LO/2, HDL Counter/2
  HDL Counter1/1 -> CC4/1, CC3/1
  CC1/1 -> LO1/3
  CC2/1 -> LO1/4
  CC3/1 -> LO1/1
  CC4/1 -> LO1/2
  reset/1 -> HDL Counter1/1, HDL Counter/1
  LO1/1 -> pixelBusGenerator/1(validIn)
  pixelBusGenerator/1(busOut) -> busOut/1

== system SGBMDisparity/SGBMHDLAlgorithm/SGBMHDLAlgorithmWorker/MatchingCost/CensusTransform1/zeroPadding ==
  pixelIn : Inport
  ctrlIn : Inport  Port=2
  Bus Selector : BusSelector  OutputSignals=valid,hStart,vStart
  CC5 : simulink/Logic and Bit Operations/Compare To Constant  relop===  const=1  OutDataTypeStr=boolean
  Constant : Constant  Value=0  VectorParams1D=off  OutDataTypeStr=uint8  SampleTime=-1
  Delay{,1..6,14} (8 alike) : Delay  DelayLength=1
  FIFO : Subsystem
  HDLC3 : hdlsllib/Sources/HDL Counter  CountType=Count limited  CountInit=0  CountStep=1  CountMax=3  CountFromType=Initial value  CountFrom=0  CountResetPort=on  CountLoadPort=off  CountEnbPort=on  CountDirPort=off  CountHitOutputPort=off  CountDataType=Unsigned  CountWordLen=2  CountFracLen=0  CountSampTime=1
  Logical Operator : Logic  Operator=OR  AllPortsSameDT=off  OutDataTypeStr=boolean
  Logical Operator1 : Logic  AllPortsSameDT=off  OutDataTypeStr=boolean
  Logical Operator2 : Logic  AllPortsSameDT=off  OutDataTypeStr=boolean
  Logical Operator3 : Logic  Operator=NOT  AllPortsSameDT=off  OutDataTypeStr=boolean
  Logical Operator4 : Logic  Operator=OR  Inputs=3  AllPortsSameDT=off  OutDataTypeStr=boolean
  Logical Operator5 : Logic  AllPortsSameDT=off  OutDataTypeStr=boolean
  Switch : Switch  Criteria=u2 ~= 0  ZeroCross=off
  popSubsystem : Subsystem
  pixelOut : Outport  VectorParamsAs1DForOutWhenUnconnected=off
  validOut : Outport  Port=2  VectorParamsAs1DForOutWhenUnconnected=off
  resetOut : Outport  Port=3  VectorParamsAs1DForOutWhenUnconnected=off
  wires:
  FIFO/1(dataOut) -> Switch/1
  Bus Selector/2 -> Delay4/1  "<hStart>"
  Bus Selector/3 -> resetOut/1, Logical Operator4/1, FIFO/4(Reset), Logical Operator/2, Delay5/1  "<vStart>"
  Switch/1 -> pixelOut/1
  FIFO/2(empty) -> Logical Operator3/1
  Bus Selector/1 -> Delay/1  "<valid>"
  Delay1/1 -> validOut/1
  Delay14/1 -> Switch/2
  Constant/1 -> Switch/3
  ctrlIn/1 -> Bus Selector/1
  pixelIn/1 -> Delay3/1
  Logical Operator2/1 -> FIFO/3(Pop), Delay14/1
  popSubsystem/2(pop) -> Logical Operator2/1
  Logical Operator4/1 -> Logical Operator5/1, popSubsystem/Enable
  Logical Operator3/1 -> Logical Operator4/2, Logical Operator2/2
  popSubsystem/3(lastRowOut) -> Delay2/1
  Logical Operator5/1 -> Delay1/1
  HDLC3/1 -> CC5/1
  Logical Operator1/1 -> HDLC3/2
  CC5/1 -> Logical Operator5/2, popSubsystem/1(enable)
  Delay2/1 -> Logical Operator4/3
  Delay/1 -> FIFO/2(Push)
  Delay3/1 -> FIFO/1(dataIn)
  Delay4/1 -> Logical Operator1/1
  Logical Operator/1 -> popSubsystem/2(reset), HDLC3/1
  popSubsystem/1(done) -> Delay6/1
  Delay5/1 -> Logical Operator1/2
  Delay6/1 -> Logical Operator/1

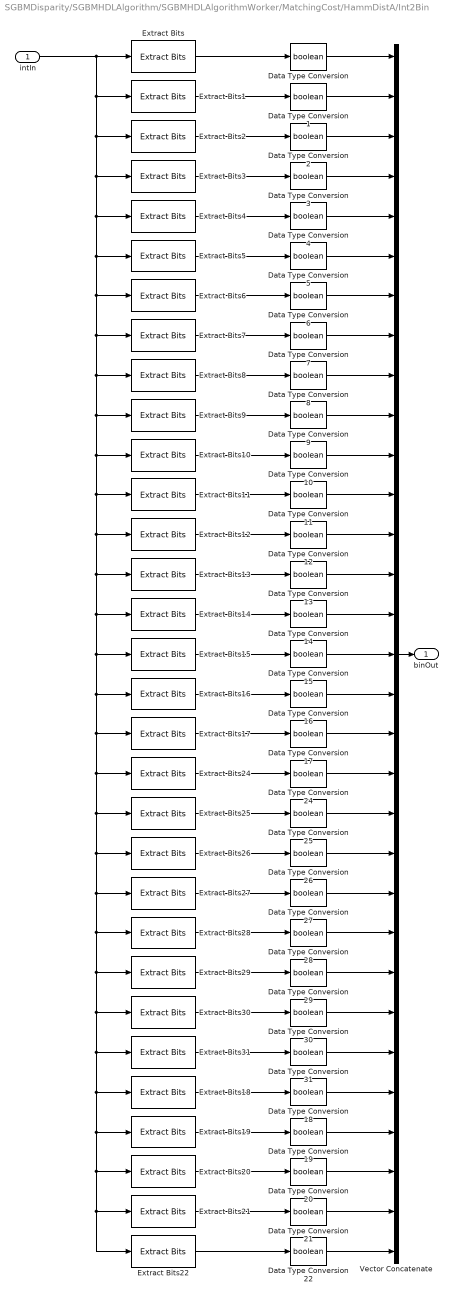
== system SGBMDisparity/SGBMHDLAlgorithm/SGBMHDLAlgorithmWorker/MatchingCost/HammDistA/Int2Bin ==
  intIn : Inport
  Data Type Conversion{,1..22,24..31} (31 alike) : DataTypeConversion  OutDataTypeStr=boolean
  Extract Bits : simulink/Logic and Bit Operations/Extract Bits  bitsToExtract=Range of bits  numBits=8  bitIdxRange=[30]  outScalingMode=Treat bit field as an integer
  Extract Bits1 : simulink/Logic and Bit Operations/Extract Bits  bitsToExtract=Range of bits  numBits=8  bitIdxRange=[29]  outScalingMode=Treat bit field as an integer
  Extract Bits10 : simulink/Logic and Bit Operations/Extract Bits  bitsToExtract=Range of bits  numBits=8  bitIdxRange=[20]  outScalingMode=Preserve fixed-point scaling
  Extract Bits11 : simulink/Logic and Bit Operations/Extract Bits  bitsToExtract=Range of bits  numBits=8  bitIdxRange=[19]  outScalingMode=Preserve fixed-point scaling
  Extract Bits12 : simulink/Logic and Bit Operations/Extract Bits  bitsToExtract=Range of bits  numBits=8  bitIdxRange=[18]  outScalingMode=Preserve fixed-point scaling
  Extract Bits13 : simulink/Logic and Bit Operations/Extract Bits  bitsToExtract=Range of bits  numBits=8  bitIdxRange=[17]  outScalingMode=Preserve fixed-point scaling
  Extract Bits14 : simulink/Logic and Bit Operations/Extract Bits  bitsToExtract=Range of bits  numBits=8  bitIdxRange=[16]  outScalingMode=Preserve fixed-point scaling
  Extract Bits15 : simulink/Logic and Bit Operations/Extract Bits  bitsToExtract=Range of bits  numBits=8  bitIdxRange=[15]  outScalingMode=Preserve fixed-point scaling
  Extract Bits16 : simulink/Logic and Bit Operations/Extract Bits  bitsToExtract=Range of bits  numBits=8  bitIdxRange=[14]  outScalingMode=Preserve fixed-point scaling
  Extract Bits17 : simulink/Logic and Bit Operations/Extract Bits  bitsToExtract=Range of bits  numBits=8  bitIdxRange=[13]  outScalingMode=Preserve fixed-point scaling
  Extract Bits18 : simulink/Logic and Bit Operations/Extract Bits  bitsToExtract=Range of bits  numBits=8  bitIdxRange=[4]  outScalingMode=Preserve fixed-point scaling
  Extract Bits19 : simulink/Logic and Bit Operations/Extract Bits  bitsToExtract=Range of bits  numBits=8  bitIdxRange=[3]  outScalingMode=Preserve fixed-point scaling
  Extract Bits2 : simulink/Logic and Bit Operations/Extract Bits  bitsToExtract=Range of bits  numBits=8  bitIdxRange=[28]  outScalingMode=Treat bit field as an integer
  Extract Bits20 : simulink/Logic and Bit Operations/Extract Bits  bitsToExtract=Range of bits  numBits=8  bitIdxRange=[2]  outScalingMode=Preserve fixed-point scaling
  Extract Bits21 : simulink/Logic and Bit Operations/Extract Bits  bitsToExtract=Range of bits  numBits=8  bitIdxRange=[1]  outScalingMode=Preserve fixed-point scaling
  Extract Bits22 : simulink/Logic and Bit Operations/Extract Bits  bitsToExtract=Range of bits  numBits=8  bitIdxRange=[0]  outScalingMode=Preserve fixed-point scaling
  Extract Bits24 : simulink/Logic and Bit Operations/Extract Bits  bitsToExtract=Range of bits  numBits=8  bitIdxRange=[12]  outScalingMode=Preserve fixed-point scaling
  Extract Bits25 : simulink/Logic and Bit Operations/Extract Bits  bitsToExtract=Range of bits  numBits=8  bitIdxRange=[11]  outScalingMode=Preserve fixed-point scaling
  Extract Bits26 : simulink/Logic and Bit Operations/Extract Bits  bitsToExtract=Range of bits  numBits=8  bitIdxRange=[10]  outScalingMode=Preserve fixed-point scaling
  Extract Bits27 : simulink/Logic and Bit Operations/Extract Bits  bitsToExtract=Range of bits  numBits=8  bitIdxRange=[9]  outScalingMode=Preserve fixed-point scaling
  Extract Bits28 : simulink/Logic and Bit Operations/Extract Bits  bitsToExtract=Range of bits  numBits=8  bitIdxRange=[8]  outScalingMode=Preserve fixed-point scaling
  Extract Bits29 : simulink/Logic and Bit Operations/Extract Bits  bitsToExtract=Range of bits  numBits=8  bitIdxRange=[7]  outScalingMode=Preserve fixed-point scaling
  Extract Bits3 : simulink/Logic and Bit Operations/Extract Bits  bitsToExtract=Range of bits  numBits=8  bitIdxRange=[27]  outScalingMode=Treat bit field as an integer
  Extract Bits30 : simulink/Logic and Bit Operations/Extract Bits  bitsToExtract=Range of bits  numBits=8  bitIdxRange=[6]  outScalingMode=Preserve fixed-point scaling
  Extract Bits31 : simulink/Logic and Bit Operations/Extract Bits  bitsToExtract=Range of bits  numBits=8  bitIdxRange=[5]  outScalingMode=Preserve fixed-point scaling
  Extract Bits4 : simulink/Logic and Bit Operations/Extract Bits  bitsToExtract=Range of bits  numBits=8  bitIdxRange=[26]  outScalingMode=Treat bit field as an integer
  Extract Bits5 : simulink/Logic and Bit Operations/Extract Bits  bitsToExtract=Range of bits  numBits=8  bitIdxRange=[25]  outScalingMode=Treat bit field as an integer
  Extract Bits6 : simulink/Logic and Bit Operations/Extract Bits  bitsToExtract=Range of bits  numBits=8  bitIdxRange=[24]  outScalingMode=Treat bit field as an integer
  Extract Bits7 : simulink/Logic and Bit Operations/Extract Bits  bitsToExtract=Range of bits  numBits=8  bitIdxRange=[23]  outScalingMode=Treat bit field as an integer
  Extract Bits8 : simulink/Logic and Bit Operations/Extract Bits  bitsToExtract=Range of bits  numBits=8  bitIdxRange=[22]  outScalingMode=Preserve fixed-point scaling
  Extract Bits9 : simulink/Logic and Bit Operations/Extract Bits  bitsToExtract=Range of bits  numBits=8  bitIdxRange=[21]  outScalingMode=Preserve fixed-point scaling
  Vector Concatenate : Concatenate  NumInputs=31
  binOut : Outport  VectorParamsAs1DForOutWhenUnconnected=off
  wires:
  Extract Bits6/1 -> Data Type Conversion6/1
  Extract Bits8/1 -> Data Type Conversion8/1
  Extract Bits1/1 -> Data Type Conversion1/1
  Extract Bits2/1 -> Data Type Conversion2/1
  Extract Bits9/1 -> Data Type Conversion9/1
  Extract Bits10/1 -> Data Type Conversion10/1
  Extract Bits3/1 -> Data Type Conversion3/1
  Extract Bits4/1 -> Data Type Conversion4/1
  Extract Bits11/1 -> Data Type Conversion11/1
  Extract Bits12/1 -> Data Type Conversion12/1
  Extract Bits13/1 -> Data Type Conversion13/1
  Extract Bits/1 -> Data Type Conversion/1
  Extract Bits7/1 -> Data Type Conversion7/1
  Extract Bits5/1 -> Data Type Conversion5/1
  Extract Bits31/1 -> Data Type Conversion31/1
  Extract Bits26/1 -> Data Type Conversion26/1
  Extract Bits18/1 -> Data Type Conversion18/1
  Extract Bits14/1 -> Data Type Conversion14/1
  Extract Bits21/1 -> Data Type Conversion21/1
  Extract Bits16/1 -> Data Type Conversion16/1
  Extract Bits25/1 -> Data Type Conversion25/1
  Extract Bits27/1 -> Data Type Conversion27/1
  Extract Bits30/1 -> Data Type Conversion30/1
  Extract Bits20/1 -> Data Type Conversion20/1
  Extract Bits28/1 -> Data Type Conversion28/1
  Extract Bits22/1 -> Data Type Conversion22/1
  Extract Bits24/1 -> Data Type Conversion24/1
  Extract Bits19/1 -> Data Type Conversion19/1
  Extract Bits15/1 -> Data Type Conversion15/1
  Extract Bits17/1 -> Data Type Conversion17/1
  Extract Bits29/1 -> Data Type Conversion29/1
  Vector Concatenate/1 -> binOut/1
  intIn/1 -> Extract Bits/1, Extract Bits1/1, Extract Bits2/1, Extract Bits3/1, Extract Bits4/1, Extract Bits5/1, Extract Bits6/1, Extract Bits7/1, Extract Bits8/1, Extract Bits9/1, Extract Bits10/1, Extract Bits11/1, Extract Bits12/1, Extract Bits13/1, Extract Bits14/1, Extract Bits15/1, Extract Bits16/1, Extract Bits17/1, Extract Bits24/1, Extract Bits25/1, Extract Bits26/1, Extract Bits27/1, Extract Bits28/1, Extract Bits29/1, Extract Bits30/1, Extract Bits31/1, Extract Bits18/1, Extract Bits19/1, Extract Bits20/1, Extract Bits21/1, Extract Bits22/1
  Data Type Conversion/1 -> Vector Concatenate/1
  Data Type Conversion1/1 -> Vector Concatenate/2
  Data Type Conversion2/1 -> Vector Concatenate/3
  Data Type Conversion3/1 -> Vector Concatenate/4
  Data Type Conversion4/1 -> Vector Concatenate/5
  Data Type Conversion7/1 -> Vector Concatenate/8
  Data Type Conversion6/1 -> Vector Concatenate/7
  Data Type Conversion5/1 -> Vector Concatenate/6
  Data Type Conversion8/1 -> Vector Concatenate/9
  Data Type Conversion10/1 -> Vector Concatenate/11
  Data Type Conversion9/1 -> Vector Concatenate/10
  Data Type Conversion11/1 -> Vector Concatenate/12
  Data Type Conversion14/1 -> Vector Concatenate/15
  Data Type Conversion12/1 -> Vector Concatenate/13
  Data Type Conversion13/1 -> Vector Concatenate/14
  Data Type Conversion15/1 -> Vector Concatenate/16
  Data Type Conversion20/1 -> Vector Concatenate/29
  Data Type Conversion21/1 -> Vector Concatenate/30
  Data Type Conversion24/1 -> Vector Concatenate/19
  Data Type Conversion22/1 -> Vector Concatenate/31
  Data Type Conversion27/1 -> Vector Concatenate/22
  Data Type Conversion26/1 -> Vector Concatenate/21
  Data Type Conversion25/1 -> Vector Concatenate/20
  Data Type Conversion29/1 -> Vector Concatenate/24
  Data Type Conversion28/1 -> Vector Concatenate/23
  Data Type Conversion30/1 -> Vector Concatenate/25
  Data Type Conversion31/1 -> Vector Concatenate/26
  Data Type Conversion16/1 -> Vector Concatenate/17
  Data Type Conversion17/1 -> Vector Concatenate/18
  Data Type Conversion19/1 -> Vector Concatenate/28
  Data Type Conversion18/1 -> Vector Concatenate/27

== system SGBMDisparity/SGBMHDLAlgorithm/SGBMHDLAlgorithmWorker/MatchingCost/HammDistA/enabledTappedDelay ==
  pixelIn : Inport
  Enable : EnablePort
  Tapped Delay : simulink/Discrete/Tapped Delay  vinit=0  samptime=-1  NumDelays=disparityLevels-1  DelayOrder=Newest  includeCurrent=on
  pixelOut : Outport  InitialOutput=0  VectorParamsAs1DForOutWhenUnconnected=off
  wires:
  Tapped Delay/1 -> pixelOut/1
  pixelIn/1 -> Tapped Delay/1
